simulink model "untitled"  (R2017b)
settings: Solver=VariableStepAuto  StartTime=0.0  StopTime=10.0  RelTol=1e-3
libraries: lib_StateEstimation x2
settings Model: Creator=ross  LastModifiedBy=ross

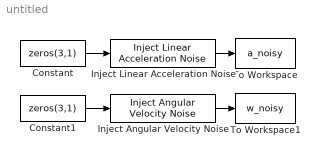
== system untitled ==
  Constant : Constant  Value=zeros(3,1)
  Constant1 : Constant  Value=zeros(3,1)
  Inject Angular Velocity Noise : lib_StateEstimation/Inject Angular Velocity Noise
  Inject Linear Acceleration Noise : lib_StateEstimation/Inject Linear Acceleration Noise
  To Workspace : ToWorkspace  VariableName=a_noisy  SaveFormat=Timeseries  SampleTime=-1
  To Workspace1 : ToWorkspace  VariableName=w_noisy  SaveFormat=Timeseries  SampleTime=-1
  wires:
  Constant/1 -> Inject Linear Acceleration Noise/1
  Inject Linear Acceleration Noise/1 -> To Workspace/1
  Constant1/1 -> Inject Angular Velocity Noise/1
  Inject Angular Velocity Noise/1 -> To Workspace1/1
